simulink model "kalman_filter_sysObj"  (R2020a)
settings: Solver=FixedStepDiscrete  StartTime=0.0  StopTime=10.0  FixedStep=dt  RelTol=1e-3  SampleTimeConstraint=STIndependent
model workspace (MAT data in the model file):
  P0 = Simulink.Parameter
  P0.Value = [1e-06  0  0; 0  1e-06  0; 0  0  1e-06]
  P0.DataType = 'auto'
  P0.Dimensions = [3 3]
  Q = Simulink.Parameter
  Q.Value = [3.49065850399e-09  0  0; 0  3.49065850399e-09  0; 0  0  3.49065850399e-09]
  Q.Description = 'Q = dt^4/4*acceleration covariance'
  Q.DataType = 'auto'
  Q.Dimensions = [3 3]
  R = Simulink.Parameter
  R.Value = [0.0174532925199  0  0; 0  0.0174532925199  0; 0  0  0.0174532925199]
  R.Description = 'sensor covariance'
  R.DataType = 'auto'
  R.Dimensions = [3 3]
  dt = Simulink.Parameter
  dt.Value = 0.02
  dt.DataType = 'double'
  dt.Dimensions = [1 1]
  nu = Simulink.Parameter
  nu.Value = [3 1]
  nu.DataType = 'auto'
  nu.Dimensions = [1 2]
  nz = Simulink.Parameter
  nz.Value = [3 1]
  nz.DataType = 'auto'
  nz.Dimensions = [1 2]
  x0 = Simulink.Parameter
  x0.Value = [0; 0; 0]
  x0.DataType = 'auto'
  x0.Dimensions = [3 1]
values from neighbouring files (symbols this model uses):
  R = diag(accel_var)    [load_tune.m]
settings Model: ParameterArgumentNames=P0,Q,R,dt,x0  OrderedModelArguments=off  Creator=Test  LastModifiedBy=Jason
settings DataIOCC: ReturnWorkspaceOutputs=off
settings DebuggingCC: AllowSymbolicDim=off  ArithmeticOperatorsInVariantConditions=warning
settings SFSimCC: SimUseLocalCustomCode=off  CustomCodeUndefinedFunction=UseInterfaceOnly
settings RTWCC: RTWUseLocalCustomCode=off

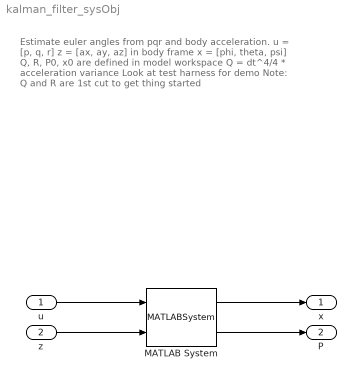
== system kalman_filter_sysObj ==
  note: Estimate euler angles from pqr and body acceleration.
      |
      | u = [p, q, r]
      | z = [ax, ay, az] in body frame
      | x = [phi, theta, psi]
      |
      | Q, R, P0, x0 are defined in model workspace
      |
      | Q = dt^4/4 * acceleration variance
      |
      | Look at test harness for demo
      |
      | Note: Q and R are 1st cut to get thing started
  u : Inport  PortDimensions=nz
  z : Inport  Port=2  PortDimensions=nz
  MATLAB System : MATLABSystem  System=EKF_Euler  Q=Q  R=R  P0=P0  x0=x0  gyroBias=[0;0;0]  accelBias=[0;0;0]  dt=dt  SimulateUsing=Code generation
      mask Type: EKF_Euler
      mask Display:
      | disp('EKF_Euler');
      | port_label('input',1,'u');
      | port_label('input',2,'z');
      | port_label('output',1,'x');
      | port_label('output',2,'P');
  x : Outport  VectorParamsAs1DForOutWhenUnconnected=off
  P : Outport  Port=2  VectorParamsAs1DForOutWhenUnconnected=off
  wires:
  MATLAB System/1 -> x/1
  MATLAB System/2 -> P/1
  u/1 -> MATLAB System/1
  z/1 -> MATLAB System/2
